simulink model "TBRe19_ECU_SequentialTests"  (R2017b)
settings: Solver=FixedStepDiscrete  StartTime=0.0  StopTime=inf  FixedStep=0.0001  RelTol=1e-3
PostLoadFcn:
  | model_init();
libraries: simulink x28
(part 14 of 22)

== system TBRe19_ECU_SequentialTests/TSSBrake/Comms_And_Data_Acquisition_Layer/MCU_CAN ==
  note: Overall Functionality:
      | Read CAN messages related to motor control unit (MCU)
  Bus Creator1 : BusCreator  Inputs=4
  CanRx1 : S-Function  FunctionName=NsiCan_Rx_J1939_Ext  Parameters=data_can,channel,msg_name,ident,ident_type,dlc,signals,is_trigger,is_SA_Masked,is_TA_Masked,is_physical,is_canfd  SFunctionDeploymentMode=off  EnableBusSupport=off  mask(MUXlink Can Rx){data_can=1;HIGH_SPEED;500Kbps;No;C:\Users\TBRe-admin\Documents\Database\TBRe19_DBC_190617.dbc;0;;;0;HIGH_SPEED;500Kbps;120 Ohm;C:\Users\TBRe-admin\Documents\Database\TBRe19_DBC_190517.dbc;0;;;0;HIGH_SPEED;1000Kbps;120 Ohm;D:\TOOLS\MUXLINK\R2011b\MUXlink\misc\BASE_CAN_MUXLAB4.dbc;0;;;0;HIGH_SPEED;500Kbps;120 Ohm;D:\TOOLS\MUXLINK\R2011b\MUXlink\misc\j1939_adapt.dbc;0;;;0;HIGH_SPEED;1000Kbps;No;D:\TOOLS\MUXLINK\R2011b\MUXlink\misc\BASE_CAN_MUXLAB4.dbc;0;;, channel=1, msg_name=HS3_Temperature_Feedback, ident=0x191AFF71, ident_type=XTD, dlc=8, signals=DC_Link_Voltage;1;32;-16;0.062500;0.000000;V;MotorTemperature;1;16;-16;1.000000;0.000000;C, is_trigger=0, is_physical=0, is_canfd=0, is_SA_Masked=1, is_TA_Masked=0}
      mask prompts: data_can "data can"; msg_name "msg name"; is_SA_Masked "J1939 SA filtering"; is_TA_Masked "J1939 TA filtering"
      mask help: Receive a frame from a CAN channel.
      mask init:
      | NsiCan_Rx_J1939_Ext_InitializationFcn();
      settings: OpenFcn=NsiCan_Rx_J1939_Ext_OpenFcn();
      mask Help:
      | eval('block=get_param(gcb, ''RTWdata'');')
      | web([docroot '\toolbox\MUXlink\html\blocks/' block.MUXlink_BlockType '.html'])
      mask Callback data_can: NsiCan_Rx_J1939_Ext_ApplyFcn(1);
      mask Callback channel: NsiCan_Rx_J1939_Ext_ApplyFcn(2);
      mask Callback msg_name: NsiCan_Rx_J1939_Ext_ApplyFcn(3);
      mask Callback ident: NsiCan_Rx_J1939_Ext_ApplyFcn(4);
      mask Callback ident_type: NsiCan_Rx_J1939_Ext_ApplyFcn(5);
      mask Callback dlc: NsiCan_Rx_J1939_Ext_ApplyFcn(6);
      mask Callback signals: NsiCan_Rx_J1939_Ext_ApplyFcn(7);
      mask Callback is_trigger: NsiCan_Rx_J1939_Ext_ApplyFcn(8);
      mask Callback is_physical: NsiCan_Rx_J1939_Ext_ApplyFcn(9);
      mask Callback is_canfd: NsiCan_Rx_J1939_Ext_ApplyFcn(10);
      mask Callback is_SA_Masked: NsiCan_Rx_J1939_Ext_ApplyFcn(11);
      mask Callback is_TA_Masked: NsiCan_Rx_J1939_Ext_ApplyFcn(12);
      mask Display: image(imread('nsi.bmp'));text(0.5, 0.3, 'J1939_PGN  HS3_Temperature_Feedbackchannel CAN1', 'horizontalAlignment', 'center', 'verticalAlignment', 'base');plot([0.05 0.05 0.05 0.05 0.05 0.05 0.05 0.05 0.05 0.05]); port_label('output',1, 'DC_Link_Voltage'); port_label('output',2, 'MotorTemperature'); port_label('output',3, 'Status');
  CanRx2 : S-Function  FunctionName=NsiCan_Rx_J1939_Ext  Parameters=data_can,channel,msg_name,ident,ident_type,dlc,signals,is_trigger,is_SA_Masked,is_TA_Masked,is_physical,is_canfd  SFunctionDeploymentMode=off  EnableBusSupport=off  mask(MUXlink Can Rx){data_can=1;HIGH_SPEED;500Kbps;No;C:\Users\TBRe-admin\Documents\Database\TBRe19_DBC_190617.dbc;0;;;0;HIGH_SPEED;500Kbps;120 Ohm;C:\Users\TBRe-admin\Documents\Database\TBRe19_DBC_190517.dbc;0;;;0;HIGH_SPEED;1000Kbps;120 Ohm;D:\TOOLS\MUXLINK\R2011b\MUXlink\misc\BASE_CAN_MUXLAB4.dbc;0;;;0;HIGH_SPEED;500Kbps;120 Ohm;D:\TOOLS\MUXLINK\R2011b\MUXlink\misc\j1939_adapt.dbc;0;;;0;HIGH_SPEED;1000Kbps;No;D:\TOOLS\MUXLINK\R2011b\MUXlink\misc\BASE_CAN_MUXLAB4.dbc;0;;, channel=1, msg_name=HD4_Debug_Temperatures_B, ident=0x192BFF71, ident_type=XTD, dlc=8, signals=Debug_Temps_Heatsink;1;24;8;1.000000;0.000000;degC, is_trigger=0, is_physical=0, is_canfd=0, is_SA_Masked=1, is_TA_Masked=0}
      mask prompts: data_can "data can"; msg_name "msg name"; is_SA_Masked "J1939 SA filtering"; is_TA_Masked "J1939 TA filtering"
      mask help: Receive a frame from a CAN channel.
      mask init:
      | NsiCan_Rx_J1939_Ext_InitializationFcn();
      settings: OpenFcn=NsiCan_Rx_J1939_Ext_OpenFcn();
      mask Help:
      | eval('block=get_param(gcb, ''RTWdata'');')
      | web([docroot '\toolbox\MUXlink\html\blocks/' block.MUXlink_BlockType '.html'])
      mask Callback data_can: NsiCan_Rx_J1939_Ext_ApplyFcn(1);
      mask Callback channel: NsiCan_Rx_J1939_Ext_ApplyFcn(2);
      mask Callback msg_name: NsiCan_Rx_J1939_Ext_ApplyFcn(3);
      mask Callback ident: NsiCan_Rx_J1939_Ext_ApplyFcn(4);
      mask Callback ident_type: NsiCan_Rx_J1939_Ext_ApplyFcn(5);
      mask Callback dlc: NsiCan_Rx_J1939_Ext_ApplyFcn(6);
      mask Callback signals: NsiCan_Rx_J1939_Ext_ApplyFcn(7);
      mask Callback is_trigger: NsiCan_Rx_J1939_Ext_ApplyFcn(8);
      mask Callback is_physical: NsiCan_Rx_J1939_Ext_ApplyFcn(9);
      mask Callback is_canfd: NsiCan_Rx_J1939_Ext_ApplyFcn(10);
      mask Callback is_SA_Masked: NsiCan_Rx_J1939_Ext_ApplyFcn(11);
      mask Callback is_TA_Masked: NsiCan_Rx_J1939_Ext_ApplyFcn(12);
      mask Display: image(imread('nsi.bmp'));text(0.5, 0.3, 'J1939_PGN  HD4_Debug_Temperatures_Bchannel CAN1', 'horizontalAlignment', 'center', 'verticalAlignment', 'base');plot([0.05 0.05 0.05 0.05 0.05 0.05 0.05 0.05 0.05 0.05]); port_label('output',1, 'Debug_Temps_Heatsink'); port_label('output',2, 'Status');
  CanRx3 : S-Function  FunctionName=NsiCan_Rx_J1939_Ext  Parameters=data_can,channel,msg_name,ident,ident_type,dlc,signals,is_trigger,is_SA_Masked,is_TA_Masked,is_physical,is_canfd  SFunctionDeploymentMode=off  EnableBusSupport=off  mask(MUXlink Can Rx){data_can=1;HIGH_SPEED;500Kbps;No;C:\Users\TBRe-admin\Documents\Database\TBRe19_DBC_190617.dbc;0;;;0;HIGH_SPEED;500Kbps;120 Ohm;C:\Users\TBRe-admin\Documents\Database\TBRe19_DBC_190517.dbc;0;;;0;HIGH_SPEED;1000Kbps;120 Ohm;D:\TOOLS\MUXLINK\R2011b\MUXlink\misc\BASE_CAN_MUXLAB4.dbc;0;;;0;HIGH_SPEED;500Kbps;120 Ohm;D:\TOOLS\MUXLINK\R2011b\MUXlink\misc\j1939_adapt.dbc;0;;;0;HIGH_SPEED;1000Kbps;No;D:\TOOLS\MUXLINK\R2011b\MUXlink\misc\BASE_CAN_MUXLAB4.dbc;0;;, channel=1, msg_name=HS1_Torque_Feedback, ident=0x1918FF71, ident_type=XTD, dlc=8, signals=Speed_Measured;1;16;-16;1.000000;0.000000;RPM, is_trigger=0, is_physical=0, is_canfd=0, is_SA_Masked=1, is_TA_Masked=0}
      mask prompts: data_can "data can"; msg_name "msg name"; is_SA_Masked "J1939 SA filtering"; is_TA_Masked "J1939 TA filtering"
      mask help: Receive a frame from a CAN channel.
      mask init:
      | NsiCan_Rx_J1939_Ext_InitializationFcn();
      settings: OpenFcn=NsiCan_Rx_J1939_Ext_OpenFcn();
      mask Help:
      | eval('block=get_param(gcb, ''RTWdata'');')
      | web([docroot '\toolbox\MUXlink\html\blocks/' block.MUXlink_BlockType '.html'])
      mask Callback data_can: NsiCan_Rx_J1939_Ext_ApplyFcn(1);
      mask Callback channel: NsiCan_Rx_J1939_Ext_ApplyFcn(2);
      mask Callback msg_name: NsiCan_Rx_J1939_Ext_ApplyFcn(3);
      mask Callback ident: NsiCan_Rx_J1939_Ext_ApplyFcn(4);
      mask Callback ident_type: NsiCan_Rx_J1939_Ext_ApplyFcn(5);
      mask Callback dlc: NsiCan_Rx_J1939_Ext_ApplyFcn(6);
      mask Callback signals: NsiCan_Rx_J1939_Ext_ApplyFcn(7);
      mask Callback is_trigger: NsiCan_Rx_J1939_Ext_ApplyFcn(8);
      mask Callback is_physical: NsiCan_Rx_J1939_Ext_ApplyFcn(9);
      mask Callback is_canfd: NsiCan_Rx_J1939_Ext_ApplyFcn(10);
      mask Callback is_SA_Masked: NsiCan_Rx_J1939_Ext_ApplyFcn(11);
      mask Callback is_TA_Masked: NsiCan_Rx_J1939_Ext_ApplyFcn(12);
      mask Display: image(imread('nsi.bmp'));text(0.5, 0.3, 'J1939_PGN  HS1_Torque_Feedbackchannel CAN1', 'horizontalAlignment', 'center', 'verticalAlignment', 'base');plot([0.05 0.05 0.05 0.05 0.05 0.05 0.05 0.05 0.05 0.05]); port_label('output',1, 'Speed_Measured'); port_label('output',2, 'Status');
  HAL_MCU : Outport
  wires:
  Bus Creator1/1 -> HAL_MCU/1  "HAL_MCU"
  CanRx1/1 -> Bus Creator1/1  "MCU_Voltage"
  CanRx1/2 -> Bus Creator1/2  "Motor_Temp"
  CanRx2/1 -> Bus Creator1/3  "MCU_Temp"
  CanRx3/1 -> Bus Creator1/4  "Motor_Speed"

== system TBRe19_ECU_SequentialTests/TSSBrake/Comms_And_Data_Acquisition_Layer/SENSOR_CAN ==
  note: Overall Functionality:
      | Read CAN messages related to vehicle sensors
  Bus Creator3 : BusCreator  Inputs=9
  CanRx1 : S-Function  FunctionName=NsiCan_Rx_Ext  Parameters=data_can,channel,msg_name,ident,ident_type,dlc,signals,is_trigger,is_physical,is_canfd,is_rxgw  SFunctionDeploymentMode=off  EnableBusSupport=off  mask(MUXlink Can Rx){data_can=1;HIGH_SPEED;500Kbps;No;C:\Users\TBRe-admin\Documents\Database\TBRe19_DBC_190617.dbc;0;;;0;HIGH_SPEED;500Kbps;120 Ohm;C:\Users\TBRe-admin\Documents\Database\TBRe19_DBC_190517.dbc;0;;;0;HIGH_SPEED;1000Kbps;120 Ohm;D:\TOOLS\MUXLINK\R2011b\MUXlink\misc\BASE_CAN_MUXLAB4.dbc;0;;;0;HIGH_SPEED;500Kbps;120 Ohm;D:\TOOLS\MUXLINK\R2011b\MUXlink\misc\j1939_adapt.dbc;0;;;0;HIGH_SPEED;1000Kbps;No;D:\TOOLS\MUXLINK\R2011b\MUXlink\misc\BASE_CAN_MUXLAB4.dbc;0;;, channel=1, msg_name=Front_Wheel_Speeds, ident=0x502, ident_type=STD, dlc=6, signals=Front_Left_Wheel_Speed;1;16;16;0.100000;0.000000;rpm;Front_Right_Wheel_Speed;1;0;16;0.100000;0.000000;rpm;Vehicle_Speed;1;32;16;0.010000;0.000000;_, is_trigger=0, is_physical=0, is_canfd=0, is_rxgw=0}
      mask prompts: data_can "data can"; msg_name "msg name"
      mask help: Receive a frame from a CAN channel.
      mask init:
      | NsiCan_Rx_Ext_InitializationFcn();
      settings: OpenFcn=NsiCan_Rx_Ext_OpenFcn();
      mask Help:
      | eval('block=get_param(gcb, ''RTWdata'');')
      | web([docroot '\toolbox\MUXlink\html\blocks/' block.MUXlink_BlockType '.html'])
      mask Callback data_can: NsiCan_Rx_Ext_ApplyFcn(1);
      mask Callback channel: NsiCan_Rx_Ext_ApplyFcn(2);
      mask Callback msg_name: NsiCan_Rx_Ext_ApplyFcn(3);
      mask Callback ident: NsiCan_Rx_Ext_ApplyFcn(4);
      mask Callback ident_type: NsiCan_Rx_Ext_ApplyFcn(5);
      mask Callback dlc: NsiCan_Rx_Ext_ApplyFcn(6);
      mask Callback signals: NsiCan_Rx_Ext_ApplyFcn(7);
      mask Callback is_trigger: NsiCan_Rx_Ext_ApplyFcn(8);
      mask Callback is_physical: NsiCan_Rx_Ext_ApplyFcn(9);
      mask Callback is_canfd: NsiCan_Rx_Ext_ApplyFcn(10);
      mask Callback is_rxgw: NsiCan_Rx_Ext_ApplyFcn(11);
      mask Display: image(imread('nsi.bmp'));text(0.5, 0.3, 'RX_Front_Wheel_Speeds_CAN1', 'horizontalAlignment', 'center', 'verticalAlignment', 'base');plot([0.05 0.05 0.05 0.05 0.05 0.05 0.05 0.05 0.05 0.05]); port_label('output',1, 'Front_Left_Wheel_Speed'); port_label('output',2, 'Front_Right_Wheel_Speed'); port_label('output',3, 'Vehicle_Speed'); port_label('output',4, 'Status');
  CanRx2 : S-Function  FunctionName=NsiCan_Rx_Ext  Parameters=data_can,channel,msg_name,ident,ident_type,dlc,signals,is_trigger,is_physical,is_canfd,is_rxgw  SFunctionDeploymentMode=off  EnableBusSupport=off  mask(MUXlink Can Rx){data_can=1;HIGH_SPEED;500Kbps;No;C:\Users\TBRe-admin\Documents\Database\TBRe19_DBC_190617.dbc;0;;;0;HIGH_SPEED;500Kbps;120 Ohm;C:\Users\TBRe-admin\Documents\Database\TBRe19_DBC_190517.dbc;0;;;0;HIGH_SPEED;1000Kbps;120 Ohm;D:\TOOLS\MUXLINK\R2011b\MUXlink\misc\BASE_CAN_MUXLAB4.dbc;0;;;0;HIGH_SPEED;500Kbps;120 Ohm;D:\TOOLS\MUXLINK\R2011b\MUXlink\misc\j1939_adapt.dbc;0;;;0;HIGH_SPEED;1000Kbps;No;D:\TOOLS\MUXLINK\R2011b\MUXlink\misc\BASE_CAN_MUXLAB4.dbc;0;;, channel=1, msg_name=Rear_Wheel_Speed, ident=0x501, ident_type=STD, dlc=6, signals=Rear_Left_Wheel_Speed;1;16;16;0.100000;0.000000;rpm;Rear_Right_Wheel_Speed;1;0;16;0.100000;0.000000;rpm;Rear_Wheel_Speed;1;32;16;0.010000;0.000000;km/h, is_trigger=0, is_physical=0, is_canfd=0, is_rxgw=0}
      mask prompts: data_can "data can"; msg_name "msg name"
      mask help: Receive a frame from a CAN channel.
      mask init:
      | NsiCan_Rx_Ext_InitializationFcn();
      settings: OpenFcn=NsiCan_Rx_Ext_OpenFcn();
      mask Help:
      | eval('block=get_param(gcb, ''RTWdata'');')
      | web([docroot '\toolbox\MUXlink\html\blocks/' block.MUXlink_BlockType '.html'])
      mask Callback data_can: NsiCan_Rx_Ext_ApplyFcn(1);
      mask Callback channel: NsiCan_Rx_Ext_ApplyFcn(2);
      mask Callback msg_name: NsiCan_Rx_Ext_ApplyFcn(3);
      mask Callback ident: NsiCan_Rx_Ext_ApplyFcn(4);
      mask Callback ident_type: NsiCan_Rx_Ext_ApplyFcn(5);
      mask Callback dlc: NsiCan_Rx_Ext_ApplyFcn(6);
      mask Callback signals: NsiCan_Rx_Ext_ApplyFcn(7);
      mask Callback is_trigger: NsiCan_Rx_Ext_ApplyFcn(8);
      mask Callback is_physical: NsiCan_Rx_Ext_ApplyFcn(9);
      mask Callback is_canfd: NsiCan_Rx_Ext_ApplyFcn(10);
      mask Callback is_rxgw: NsiCan_Rx_Ext_ApplyFcn(11);
      mask Display: image(imread('nsi.bmp'));text(0.5, 0.3, 'RX_Rear_Wheel_Speed_CAN1', 'horizontalAlignment', 'center', 'verticalAlignment', 'base');plot([0.05 0.05 0.05 0.05 0.05 0.05 0.05 0.05 0.05 0.05]); port_label('output',1, 'Rear_Left_Wheel_Speed'); port_label('output',2, 'Rear_Right_Wheel_Speed'); port_label('output',3, 'Rear_Wheel_Speed'); port_label('output',4, 'Status');
  CanRx5 : S-Function  FunctionName=NsiCan_Rx_Ext  Parameters=data_can,channel,msg_name,ident,ident_type,dlc,signals,is_trigger,is_physical,is_canfd,is_rxgw  SFunctionDeploymentMode=off  EnableBusSupport=off  mask(MUXlink Can Rx){data_can=1;HIGH_SPEED;500Kbps;No;C:\Users\TBRe-admin\Documents\Database\TBRe19_DBC_190617.dbc;0;;;0;HIGH_SPEED;500Kbps;120 Ohm;C:\Users\TBRe-admin\Documents\Database\TBRe19_DBC_190517.dbc;0;;;0;HIGH_SPEED;1000Kbps;120 Ohm;D:\TOOLS\MUXLINK\R2011b\MUXlink\misc\BASE_CAN_MUXLAB4.dbc;0;;;0;HIGH_SPEED;500Kbps;120 Ohm;D:\TOOLS\MUXLINK\R2011b\MUXlink\misc\j1939_adapt.dbc;0;;;0;HIGH_SPEED;1000Kbps;No;D:\TOOLS\MUXLINK\R2011b\MUXlink\misc\BASE_CAN_MUXLAB4.dbc;0;;, channel=1, msg_name=SteeringWheelSensor, ident=0x234, ident_type=STD, dlc=5, signals=Acc_Angle;1;0;-16;0.100000;0.000000;Degrees, is_trigger=0, is_physical=0, is_canfd=0, is_rxgw=0}
      mask prompts: data_can "data can"; msg_name "msg name"
      mask help: Receive a frame from a CAN channel.
      mask init:
      | NsiCan_Rx_Ext_InitializationFcn();
      settings: OpenFcn=NsiCan_Rx_Ext_OpenFcn();
      mask Help:
      | eval('block=get_param(gcb, ''RTWdata'');')
      | web([docroot '\toolbox\MUXlink\html\blocks/' block.MUXlink_BlockType '.html'])
      mask Callback data_can: NsiCan_Rx_Ext_ApplyFcn(1);
      mask Callback channel: NsiCan_Rx_Ext_ApplyFcn(2);
      mask Callback msg_name: NsiCan_Rx_Ext_ApplyFcn(3);
      mask Callback ident: NsiCan_Rx_Ext_ApplyFcn(4);
      mask Callback ident_type: NsiCan_Rx_Ext_ApplyFcn(5);
      mask Callback dlc: NsiCan_Rx_Ext_ApplyFcn(6);
      mask Callback signals: NsiCan_Rx_Ext_ApplyFcn(7);
      mask Callback is_trigger: NsiCan_Rx_Ext_ApplyFcn(8);
      mask Callback is_physical: NsiCan_Rx_Ext_ApplyFcn(9);
      mask Callback is_canfd: NsiCan_Rx_Ext_ApplyFcn(10);
      mask Callback is_rxgw: NsiCan_Rx_Ext_ApplyFcn(11);
      mask Display: image(imread('nsi.bmp'));text(0.5, 0.3, 'RX_SteeringWheelSensor_CAN1', 'horizontalAlignment', 'center', 'verticalAlignment', 'base');plot([0.05 0.05 0.05 0.05 0.05 0.05 0.05 0.05 0.05 0.05]); port_label('output',1, 'Acc_Angle'); port_label('output',2, 'Status');
  CanRx8 : S-Function  FunctionName=NsiCan_Rx_Ext  Parameters=data_can,channel,msg_name,ident,ident_type,dlc,signals,is_trigger,is_physical,is_canfd,is_rxgw  SFunctionDeploymentMode=off  EnableBusSupport=off  mask(MUXlink Can Rx){data_can=1;HIGH_SPEED;500Kbps;No;C:\Users\TBRe-admin\Documents\Database\TBRe19_DBC_190617.dbc;0;;;0;HIGH_SPEED;500Kbps;120 Ohm;C:\Users\TBRe-admin\Documents\Database\TBRe19_DBC_190517.dbc;0;;;0;HIGH_SPEED;1000Kbps;120 Ohm;D:\TOOLS\MUXLINK\R2011b\MUXlink\misc\BASE_CAN_MUXLAB4.dbc;0;;;0;HIGH_SPEED;500Kbps;120 Ohm;D:\TOOLS\MUXLINK\R2011b\MUXlink\misc\j1939_adapt.dbc;0;;;0;HIGH_SPEED;1000Kbps;No;D:\TOOLS\MUXLINK\R2011b\MUXlink\misc\BASE_CAN_MUXLAB4.dbc;0;;, channel=1, msg_name=AccelerometerY, ident=0x174, ident_type=STD, dlc=8, signals=Acc_Yaw;1;0;16;0.005000;0.000000;_, is_trigger=0, is_physical=0, is_canfd=0, is_rxgw=0}
      mask prompts: data_can "data can"; msg_name "msg name"
      mask help: Receive a frame from a CAN channel.
      mask init:
      | NsiCan_Rx_Ext_InitializationFcn();
      settings: OpenFcn=NsiCan_Rx_Ext_OpenFcn();
      mask Help:
      | eval('block=get_param(gcb, ''RTWdata'');')
      | web([docroot '\toolbox\MUXlink\html\blocks/' block.MUXlink_BlockType '.html'])
      mask Callback data_can: NsiCan_Rx_Ext_ApplyFcn(1);
      mask Callback channel: NsiCan_Rx_Ext_ApplyFcn(2);
      mask Callback msg_name: NsiCan_Rx_Ext_ApplyFcn(3);
      mask Callback ident: NsiCan_Rx_Ext_ApplyFcn(4);
      mask Callback ident_type: NsiCan_Rx_Ext_ApplyFcn(5);
      mask Callback dlc: NsiCan_Rx_Ext_ApplyFcn(6);
      mask Callback signals: NsiCan_Rx_Ext_ApplyFcn(7);
      mask Callback is_trigger: NsiCan_Rx_Ext_ApplyFcn(8);
      mask Callback is_physical: NsiCan_Rx_Ext_ApplyFcn(9);
      mask Callback is_canfd: NsiCan_Rx_Ext_ApplyFcn(10);
      mask Callback is_rxgw: NsiCan_Rx_Ext_ApplyFcn(11);
      mask Display: image(imread('nsi.bmp'));text(0.5, 0.3, 'RX_AccelerometerY_CAN1', 'horizontalAlignment', 'center', 'verticalAlignment', 'base');plot([0.05 0.05 0.05 0.05 0.05 0.05 0.05 0.05 0.05 0.05]); port_label('output',1, 'Acc_Yaw'); port_label('output',2, 'Status');
  CanRx9 : S-Function  FunctionName=NsiCan_Rx_Ext  Parameters=data_can,channel,msg_name,ident,ident_type,dlc,signals,is_trigger,is_physical,is_canfd,is_rxgw  SFunctionDeploymentMode=off  EnableBusSupport=off  mask(MUXlink Can Rx){data_can=1;HIGH_SPEED;500Kbps;No;C:\Users\TBRe-admin\Documents\Database\TBRe19_DBC_190620.dbc;0;;;0;HIGH_SPEED;500Kbps;120 Ohm;C:\Users\TBRe-admin\Documents\Database\TBRe19_DBC_190517.dbc;0;;;0;HIGH_SPEED;1000Kbps;120 Ohm;D:\TOOLS\MUXLINK\R2011b\MUXlink\misc\BASE_CAN_MUXLAB4.dbc;0;;;0;HIGH_SPEED;500Kbps;120 Ohm;D:\TOOLS\MUXLINK\R2011b\MUXlink\misc\j1939_adapt.dbc;0;;;0;HIGH_SPEED;1000Kbps;No;D:\TOOLS\MUXLINK\R2011b\MUXlink\misc\BASE_CAN_MUXLAB4.dbc;0;;, channel=1, msg_name=Shutdown_Data, ident=0x705, ident_type=STD, dlc=3, signals=Fault_CarShutdown;1;0;1;1.000000;0.000000;_, is_trigger=0, is_physical=0, is_canfd=0, is_rxgw=0}
      mask prompts: data_can "data can"; msg_name "msg name"
      mask help: Receive a frame from a CAN channel.
      mask init:
      | NsiCan_Rx_Ext_InitializationFcn();
      settings: OpenFcn=NsiCan_Rx_Ext_OpenFcn();
      mask Help:
      | eval('block=get_param(gcb, ''RTWdata'');')
      | web([docroot '\toolbox\MUXlink\html\blocks/' block.MUXlink_BlockType '.html'])
      mask Callback data_can: NsiCan_Rx_Ext_ApplyFcn(1);
      mask Callback channel: NsiCan_Rx_Ext_ApplyFcn(2);
      mask Callback msg_name: NsiCan_Rx_Ext_ApplyFcn(3);
      mask Callback ident: NsiCan_Rx_Ext_ApplyFcn(4);
      mask Callback ident_type: NsiCan_Rx_Ext_ApplyFcn(5);
      mask Callback dlc: NsiCan_Rx_Ext_ApplyFcn(6);
      mask Callback signals: NsiCan_Rx_Ext_ApplyFcn(7);
      mask Callback is_trigger: NsiCan_Rx_Ext_ApplyFcn(8);
      mask Callback is_physical: NsiCan_Rx_Ext_ApplyFcn(9);
      mask Callback is_canfd: NsiCan_Rx_Ext_ApplyFcn(10);
      mask Callback is_rxgw: NsiCan_Rx_Ext_ApplyFcn(11);
      mask Display: image(imread('nsi.bmp'));text(0.5, 0.3, 'RX_Shutdown_Data_CAN1', 'horizontalAlignment', 'center', 'verticalAlignment', 'base');plot([0.05 0.05 0.05 0.05 0.05 0.05 0.05 0.05 0.05 0.05]); port_label('output',1, 'Fault_CarShutdown'); port_label('output',2, 'Status');
  Sensor_Data : Outport
  wires:
  CanRx5/2 -> ?
  CanRx1/4 -> ?
  CanRx2/4 -> ?
  CanRx8/2 -> ?
  CanRx9/2 -> ?
  CanRx9/1 -> Bus Creator3/9  "Shutdown_Error"
  CanRx2/2 -> Bus Creator3/5  "Rear_Right_Wheel_Speed"
  CanRx2/3 -> Bus Creator3/6  "Rear_Wheel_Speed"
  CanRx5/1 -> Bus Creator3/7  "Steering_Angle"
  CanRx8/1 -> Bus Creator3/8  "Yaw"
  CanRx1/1 -> Bus Creator3/1  "Front_Left_Wheel_Speed"
  CanRx1/2 -> Bus Creator3/2  "Front_Right_Wheel_Speed"
  CanRx2/1 -> Bus Creator3/4  "Rear_Left_Wheel_Speed"
  Bus Creator3/1 -> Sensor_Data/1  "Sensor_Data"
  CanRx1/3 -> Bus Creator3/3  "Vehicle_Speed"

== system TBRe19_ECU_SequentialTests/TSSBrake/Comms_And_Data_Output_Layer/Hardwired_Ouputs ==
  note: Turns the MCU on
  PostPL_Data : Inport
  Bus Selector : BusSelector  OutputSignals=Hardwired_Peripherals.TSS
  DigitalOutput2 : S-Function  FunctionName=NsiIo_DigitalOutput  Parameters=channel,side,feedback  SFunctionDeploymentMode=off  EnableBusSupport=off  mask(MUXlink I/O Digital Output){channel=1, side=High, feedback=off}
      mask prompts: channel "Channel ?"; side "Side ?"; feedback "With feedback ?"
      mask help: Write Digital Output onto I/O channel.
      mask init:
      | NsiIo_DigitalOutput_InitializationFcn();
      settings: OpenFcn=NsiIo_DigitalOutput_OpenFcn();
      mask Help:
      | eval('block=get_param(gcb, ''RTWdata'');')
      | web([docroot '\toolbox\MUXlink\html\blocks/' block.MUXlink_BlockType '.html'])
      mask Callback channel: NsiIo_DigitalOutput_ApplyFcn(1);
      mask TypeOptions side: High | Low
      mask Callback side: NsiIo_DigitalOutput_ApplyFcn(2);
      mask Callback feedback: NsiIo_DigitalOutput_ApplyFcn(3);
      mask Display: image(imread('nsi.bmp'));text(0.5, 0.2, 'DigitalOutput_1', 'horizontalAlignment', 'center', 'verticalAlignment', 'base');plot([0.05 0.05 0.05 0.05 0.05 0.05 0.05 0.05 0.05 0.05]);port_label('input', 1, 'G2 : High Side');
  wires:
  PostPL_Data/1 -> Bus Selector/1
  Bus Selector/1 -> DigitalOutput2/1  "<TSS>"

== system TBRe19_ECU_SequentialTests/TSSBrake/Post_Processing_Layer/Hardwired_Peripherals ==
  note: Talk to Wilkins about when you want pump and fans
      | power switching between Vicor and LV to occur
  VFL_Data : Inport
  Bus Creator : BusCreator  Inputs=7
  Bus Selector3 : BusSelector  OutputSignals=VOM_Data.TSS
  Hardwired_Peripherals : Outport
  wires:
  VFL_Data/1 -> Bus Selector3/1
  Bus Selector3/1 -> Bus Creator/3  "<TSS>"
  Bus Creator/1 -> Hardwired_Peripherals/1  "Hardwired_Peripherals"

== system TBRe19_ECU_SequentialTests/TSSBrake/Vehicle_Functionality_Layer/Vehicle_Operation_Mode ==
  PrePL_Data : Inport
  Bus Creator : BusCreator  Inputs=5
  TSS : Subsystem
  VOM_Data : Outport
  wires:
  Bus Creator/1 -> VOM_Data/1  "Vehicle_Operation_Data"
  PrePL_Data/1 -> TSS/1(PrePL_Data)
  TSS/1(TS_StartUp) -> Bus Creator/5  "TSS"

== system TBRe19_ECU_SequentialTests/DriveFunction/Comms_And_Data_Acquisition_Layer/Hardwired_Inputs_2019/AIRs ==
  DigitalInput : S-Function  FunctionName=NsiIo_DigitalInput  Parameters=channel,is_trigger,typeof_trigger,is_wakeup,wakeup_level  SFunctionDeploymentMode=off  EnableBusSupport=off  mask(MUXlink I/O Digital Input){channel=1, is_trigger=off, typeof_trigger=Either, is_wakeup=off, wakeup_level=Low level}
      mask prompts: channel "Channel ?"; is_trigger "Trigger ?"; typeof_trigger "Type of Trigger ?"; is_wakeup "Wake-up ?"; wakeup_level "Wake-up level ?"
      mask help: Read digital input from I/O channel.
      mask init:
      | NsiIo_DigitalInput_InitializationFcn();
      settings: OpenFcn=NsiIo_DigitalInput_OpenFcn();
      mask Help:
      | eval('block=get_param(gcb, ''RTWdata'');')
      | web([docroot '\toolbox\MUXlink\html\blocks/' block.MUXlink_BlockType '.html'])
      mask Callback channel: NsiIo_DigitalInput_ApplyFcn(1);
      mask Callback is_trigger: NsiIo_DigitalInput_ApplyFcn(2);
      mask TypeOptions typeof_trigger: Rising | Falling | Either
      mask Callback typeof_trigger: NsiIo_DigitalInput_ApplyFcn(3);
      mask Callback is_wakeup: NsiIo_DigitalInput_ApplyFcn(4);
      mask TypeOptions wakeup_level: Low level | High level
      mask Callback wakeup_level: NsiIo_DigitalInput_ApplyFcn(5);
      mask Display: image(imread('nsi.bmp'));text(0.5, 0.2, 'DigitalInput_1', 'horizontalAlignment', 'center', 'verticalAlignment', 'base');plot([0.05 0.05 0.05 0.05 0.05 0.05 0.05 0.05 0.05 0.05]);port_label('output', 1, 'Ground : A1');
  DigitalInput5 : S-Function  FunctionName=NsiIo_DigitalInput  Parameters=channel,is_trigger,typeof_trigger,is_wakeup,wakeup_level  SFunctionDeploymentMode=off  EnableBusSupport=off  mask(MUXlink I/O Digital Input){channel=2, is_trigger=off, typeof_trigger=Either, is_wakeup=off, wakeup_level=Low level}
      mask prompts: channel "Channel ?"; is_trigger "Trigger ?"; typeof_trigger "Type of Trigger ?"; is_wakeup "Wake-up ?"; wakeup_level "Wake-up level ?"
      mask help: Read digital input from I/O channel.
      mask init:
      | NsiIo_DigitalInput_InitializationFcn();
      settings: OpenFcn=NsiIo_DigitalInput_OpenFcn();
      mask Help:
      | eval('block=get_param(gcb, ''RTWdata'');')
      | web([docroot '\toolbox\MUXlink\html\blocks/' block.MUXlink_BlockType '.html'])
      mask Callback channel: NsiIo_DigitalInput_ApplyFcn(1);
      mask Callback is_trigger: NsiIo_DigitalInput_ApplyFcn(2);
      mask TypeOptions typeof_trigger: Rising | Falling | Either
      mask Callback typeof_trigger: NsiIo_DigitalInput_ApplyFcn(3);
      mask Callback is_wakeup: NsiIo_DigitalInput_ApplyFcn(4);
      mask TypeOptions wakeup_level: Low level | High level
      mask Callback wakeup_level: NsiIo_DigitalInput_ApplyFcn(5);
      mask Display: image(imread('nsi.bmp'));text(0.5, 0.2, 'DigitalInput_2', 'horizontalAlignment', 'center', 'verticalAlignment', 'base');plot([0.05 0.05 0.05 0.05 0.05 0.05 0.05 0.05 0.05 0.05]);port_label('output', 1, 'Ground : A2');
  UsbTx1 : S-Function  FunctionName=NsiUsb_Tx  Parameters=signame,resolution,offset,unite  SFunctionDeploymentMode=off  EnableBusSupport=off  mask(MUXlink Usb Tx){signame=AIRLow, resolution=1, offset=0, unite=Bool}
      mask prompts: signame "Signal name ?"; resolution "Resolution ?"; offset "Offset ?"; unite "Unit ?"
      mask help: Transmit a frame on the USB Channel.
      mask init:
      | NsiUsb_Tx_InitializationFcn();
      settings: OpenFcn=NsiUsb_Tx_OpenFcn();
      mask Help:
      | eval('block=get_param(gcb, ''RTWdata'');')
      | web([docroot '\toolbox\MUXlink\html\blocks/' block.MUXlink_BlockType '.html'])
      mask Callback signame: NsiUsb_Tx_ApplyFcn(1);
      mask Callback resolution: NsiUsb_Tx_ApplyFcn(2);
      mask Callback offset: NsiUsb_Tx_ApplyFcn(3);
      mask Callback unite: NsiUsb_Tx_ApplyFcn(4);
      mask Display: image(imread('nsi.bmp'));text(0.5, 0.2, 'USB Tx', 'horizontalAlignment', 'center', 'verticalAlignment', 'base');plot([0.05 0.05 0.05 0.05 0.05 0.05 0.05 0.05 0.05 0.05]);port_label('input',1, 'AIRLow');
  UsbTx2 : S-Function  FunctionName=NsiUsb_Tx  Parameters=signame,resolution,offset,unite  SFunctionDeploymentMode=off  EnableBusSupport=off  mask(MUXlink Usb Tx){signame=AIRHigh, resolution=1, offset=0, unite=Bool}
      mask prompts: signame "Signal name ?"; resolution "Resolution ?"; offset "Offset ?"; unite "Unit ?"
      mask help: Transmit a frame on the USB Channel.
      mask init:
      | NsiUsb_Tx_InitializationFcn();
      settings: OpenFcn=NsiUsb_Tx_OpenFcn();
      mask Help:
      | eval('block=get_param(gcb, ''RTWdata'');')
      | web([docroot '\toolbox\MUXlink\html\blocks/' block.MUXlink_BlockType '.html'])
      mask Callback signame: NsiUsb_Tx_ApplyFcn(1);
      mask Callback resolution: NsiUsb_Tx_ApplyFcn(2);
      mask Callback offset: NsiUsb_Tx_ApplyFcn(3);
      mask Callback unite: NsiUsb_Tx_ApplyFcn(4);
      mask Display: image(imread('nsi.bmp'));text(0.5, 0.2, 'USB Tx', 'horizontalAlignment', 'center', 'verticalAlignment', 'base');plot([0.05 0.05 0.05 0.05 0.05 0.05 0.05 0.05 0.05 0.05]);port_label('input',1, 'AIRHigh');
  AIRLow : Outport
  AIRHigh : Outport  Port=2
  wires:
  DigitalInput/1 -> UsbTx1/1, AIRLow/1  "AIRLow"
  DigitalInput5/1 -> UsbTx2/1, AIRHigh/1  "AIRHigh"

== system TBRe19_ECU_SequentialTests/DriveFunction/Comms_And_Data_Acquisition_Layer/Hardwired_Inputs_2019/BMS ==
  DigitalInput1 : S-Function  FunctionName=NsiIo_DigitalInput  Parameters=channel,is_trigger,typeof_trigger,is_wakeup,wakeup_level  SFunctionDeploymentMode=off  EnableBusSupport=off  mask(MUXlink I/O Digital Input){channel=16, is_trigger=off, typeof_trigger=Either, is_wakeup=off, wakeup_level=Low level}
      mask prompts: channel "Channel ?"; is_trigger "Trigger ?"; typeof_trigger "Type of Trigger ?"; is_wakeup "Wake-up ?"; wakeup_level "Wake-up level ?"
      mask help: Read digital input from I/O channel.
      mask init:
      | NsiIo_DigitalInput_InitializationFcn();
      settings: OpenFcn=NsiIo_DigitalInput_OpenFcn();
      mask Help:
      | eval('block=get_param(gcb, ''RTWdata'');')
      | web([docroot '\toolbox\MUXlink\html\blocks/' block.MUXlink_BlockType '.html'])
      mask Callback channel: NsiIo_DigitalInput_ApplyFcn(1);
      mask Callback is_trigger: NsiIo_DigitalInput_ApplyFcn(2);
      mask TypeOptions typeof_trigger: Rising | Falling | Either
      mask Callback typeof_trigger: NsiIo_DigitalInput_ApplyFcn(3);
      mask Callback is_wakeup: NsiIo_DigitalInput_ApplyFcn(4);
      mask TypeOptions wakeup_level: Low level | High level
      mask Callback wakeup_level: NsiIo_DigitalInput_ApplyFcn(5);
      mask Display: image(imread('nsi.bmp'));text(0.5, 0.2, 'DigitalInput_16', 'horizontalAlignment', 'center', 'verticalAlignment', 'base');plot([0.05 0.05 0.05 0.05 0.05 0.05 0.05 0.05 0.05 0.05]);port_label('output', 1, 'Battery : H2');
  DigitalInput2 : S-Function  FunctionName=NsiIo_DigitalInput  Parameters=channel,is_trigger,typeof_trigger,is_wakeup,wakeup_level  SFunctionDeploymentMode=off  EnableBusSupport=off  mask(MUXlink I/O Digital Input){channel=17, is_trigger=off, typeof_trigger=Either, is_wakeup=off, wakeup_level=Low level}
      mask prompts: channel "Channel ?"; is_trigger "Trigger ?"; typeof_trigger "Type of Trigger ?"; is_wakeup "Wake-up ?"; wakeup_level "Wake-up level ?"
      mask help: Read digital input from I/O channel.
      mask init:
      | NsiIo_DigitalInput_InitializationFcn();
      settings: OpenFcn=NsiIo_DigitalInput_OpenFcn();
      mask Help:
      | eval('block=get_param(gcb, ''RTWdata'');')
      | web([docroot '\toolbox\MUXlink\html\blocks/' block.MUXlink_BlockType '.html'])
      mask Callback channel: NsiIo_DigitalInput_ApplyFcn(1);
      mask Callback is_trigger: NsiIo_DigitalInput_ApplyFcn(2);
      mask TypeOptions typeof_trigger: Rising | Falling | Either
      mask Callback typeof_trigger: NsiIo_DigitalInput_ApplyFcn(3);
      mask Callback is_wakeup: NsiIo_DigitalInput_ApplyFcn(4);
      mask TypeOptions wakeup_level: Low level | High level
      mask Callback wakeup_level: NsiIo_DigitalInput_ApplyFcn(5);
      mask Display: image(imread('nsi.bmp'));text(0.5, 0.2, 'DigitalInput_17', 'horizontalAlignment', 'center', 'verticalAlignment', 'base');plot([0.05 0.05 0.05 0.05 0.05 0.05 0.05 0.05 0.05 0.05]);port_label('output', 1, 'Battery : H3');
  DigitalInput6 : S-Function  FunctionName=NsiIo_DigitalInput  Parameters=channel,is_trigger,typeof_trigger,is_wakeup,wakeup_level  SFunctionDeploymentMode=off  EnableBusSupport=off  mask(MUXlink I/O Digital Input){channel=18, is_trigger=off, typeof_trigger=Either, is_wakeup=off, wakeup_level=Low level}
      mask prompts: channel "Channel ?"; is_trigger "Trigger ?"; typeof_trigger "Type of Trigger ?"; is_wakeup "Wake-up ?"; wakeup_level "Wake-up level ?"
      mask help: Read digital input from I/O channel.
      mask init:
      | NsiIo_DigitalInput_InitializationFcn();
      settings: OpenFcn=NsiIo_DigitalInput_OpenFcn();
      mask Help:
      | eval('block=get_param(gcb, ''RTWdata'');')
      | web([docroot '\toolbox\MUXlink\html\blocks/' block.MUXlink_BlockType '.html'])
      mask Callback channel: NsiIo_DigitalInput_ApplyFcn(1);
      mask Callback is_trigger: NsiIo_DigitalInput_ApplyFcn(2);
      mask TypeOptions typeof_trigger: Rising | Falling | Either
      mask Callback typeof_trigger: NsiIo_DigitalInput_ApplyFcn(3);
      mask Callback is_wakeup: NsiIo_DigitalInput_ApplyFcn(4);
      mask TypeOptions wakeup_level: Low level | High level
      mask Callback wakeup_level: NsiIo_DigitalInput_ApplyFcn(5);
      mask Display: image(imread('nsi.bmp'));text(0.5, 0.2, 'DigitalInput_18', 'horizontalAlignment', 'center', 'verticalAlignment', 'base');plot([0.05 0.05 0.05 0.05 0.05 0.05 0.05 0.05 0.05 0.05]);port_label('output', 1, 'Battery : H4');
  BMS_Multi1 : Outport
  BMS_Multi2 : Outport  Port=2
  BMS_ChargeEnable : Outport  Port=3
  wires:
  DigitalInput6/1 -> BMS_Multi1/1  "BMS_Multi1"
  DigitalInput2/1 -> BMS_ChargeEnable/1  "BMS_ChargeEnable"
  DigitalInput1/1 -> BMS_Multi2/1  "BMS_Multi2"

== system TBRe19_ECU_SequentialTests/DriveFunction/Comms_And_Data_Acquisition_Layer/Hardwired_Inputs_2019/Buttons ==
  DigitalInput1 : S-Function  FunctionName=NsiIo_DigitalInput  Parameters=channel,is_trigger,typeof_trigger,is_wakeup,wakeup_level  SFunctionDeploymentMode=off  EnableBusSupport=off  mask(MUXlink I/O Digital Input){channel=5, is_trigger=off, typeof_trigger=Either, is_wakeup=off, wakeup_level=Low level}
      mask prompts: channel "Channel ?"; is_trigger "Trigger ?"; typeof_trigger "Type of Trigger ?"; is_wakeup "Wake-up ?"; wakeup_level "Wake-up level ?"
      mask help: Read digital input from I/O channel.
      mask init:
      | NsiIo_DigitalInput_InitializationFcn();
      settings: OpenFcn=NsiIo_DigitalInput_OpenFcn();
      mask Help:
      | eval('block=get_param(gcb, ''RTWdata'');')
      | web([docroot '\toolbox\MUXlink\html\blocks/' block.MUXlink_BlockType '.html'])
      mask Callback channel: NsiIo_DigitalInput_ApplyFcn(1);
      mask Callback is_trigger: NsiIo_DigitalInput_ApplyFcn(2);
      mask TypeOptions typeof_trigger: Rising | Falling | Either
      mask Callback typeof_trigger: NsiIo_DigitalInput_ApplyFcn(3);
      mask Callback is_wakeup: NsiIo_DigitalInput_ApplyFcn(4);
      mask TypeOptions wakeup_level: Low level | High level
      mask Callback wakeup_level: NsiIo_DigitalInput_ApplyFcn(5);
      mask Display: image(imread('nsi.bmp'));text(0.5, 0.2, 'DigitalInput_5', 'horizontalAlignment', 'center', 'verticalAlignment', 'base');plot([0.05 0.05 0.05 0.05 0.05 0.05 0.05 0.05 0.05 0.05]);port_label('output', 1, 'Ground : B1');
  DigitalInput2 : S-Function  FunctionName=NsiIo_DigitalInput  Parameters=channel,is_trigger,typeof_trigger,is_wakeup,wakeup_level  SFunctionDeploymentMode=off  EnableBusSupport=off  mask(MUXlink I/O Digital Input){channel=8, is_trigger=off, typeof_trigger=Either, is_wakeup=off, wakeup_level=Low level}
      mask prompts: channel "Channel ?"; is_trigger "Trigger ?"; typeof_trigger "Type of Trigger ?"; is_wakeup "Wake-up ?"; wakeup_level "Wake-up level ?"
      mask help: Read digital input from I/O channel.
      mask init:
      | NsiIo_DigitalInput_InitializationFcn();
      settings: OpenFcn=NsiIo_DigitalInput_OpenFcn();
      mask Help:
      | eval('block=get_param(gcb, ''RTWdata'');')
      | web([docroot '\toolbox\MUXlink\html\blocks/' block.MUXlink_BlockType '.html'])
      mask Callback channel: NsiIo_DigitalInput_ApplyFcn(1);
      mask Callback is_trigger: NsiIo_DigitalInput_ApplyFcn(2);
      mask TypeOptions typeof_trigger: Rising | Falling | Either
      mask Callback typeof_trigger: NsiIo_DigitalInput_ApplyFcn(3);
      mask Callback is_wakeup: NsiIo_DigitalInput_ApplyFcn(4);
      mask TypeOptions wakeup_level: Low level | High level
      mask Callback wakeup_level: NsiIo_DigitalInput_ApplyFcn(5);
      mask Display: image(imread('nsi.bmp'));text(0.5, 0.2, 'DigitalInput_8', 'horizontalAlignment', 'center', 'verticalAlignment', 'base');plot([0.05 0.05 0.05 0.05 0.05 0.05 0.05 0.05 0.05 0.05]);port_label('output', 1, 'Ground : B4');
  DigitalInput3 : S-Function  FunctionName=NsiIo_DigitalInput  Parameters=channel,is_trigger,typeof_trigger,is_wakeup,wakeup_level  SFunctionDeploymentMode=off  EnableBusSupport=off  mask(MUXlink I/O Digital Input){channel=6, is_trigger=off, typeof_trigger=Either, is_wakeup=off, wakeup_level=Low level}
      mask prompts: channel "Channel ?"; is_trigger "Trigger ?"; typeof_trigger "Type of Trigger ?"; is_wakeup "Wake-up ?"; wakeup_level "Wake-up level ?"
      mask help: Read digital input from I/O channel.
      mask init:
      | NsiIo_DigitalInput_InitializationFcn();
      settings: OpenFcn=NsiIo_DigitalInput_OpenFcn();
      mask Help:
      | eval('block=get_param(gcb, ''RTWdata'');')
      | web([docroot '\toolbox\MUXlink\html\blocks/' block.MUXlink_BlockType '.html'])
      mask Callback channel: NsiIo_DigitalInput_ApplyFcn(1);
      mask Callback is_trigger: NsiIo_DigitalInput_ApplyFcn(2);
      mask TypeOptions typeof_trigger: Rising | Falling | Either
      mask Callback typeof_trigger: NsiIo_DigitalInput_ApplyFcn(3);
      mask Callback is_wakeup: NsiIo_DigitalInput_ApplyFcn(4);
      mask TypeOptions wakeup_level: Low level | High level
      mask Callback wakeup_level: NsiIo_DigitalInput_ApplyFcn(5);
      mask Display: image(imread('nsi.bmp'));text(0.5, 0.2, 'DigitalInput_6', 'horizontalAlignment', 'center', 'verticalAlignment', 'base');plot([0.05 0.05 0.05 0.05 0.05 0.05 0.05 0.05 0.05 0.05]);port_label('output', 1, 'Ground : B2');
  DigitalInput4 : S-Function  FunctionName=NsiIo_DigitalInput  Parameters=channel,is_trigger,typeof_trigger,is_wakeup,wakeup_level  SFunctionDeploymentMode=off  EnableBusSupport=off  mask(MUXlink I/O Digital Input){channel=7, is_trigger=off, typeof_trigger=Either, is_wakeup=off, wakeup_level=Low level}
      mask prompts: channel "Channel ?"; is_trigger "Trigger ?"; typeof_trigger "Type of Trigger ?"; is_wakeup "Wake-up ?"; wakeup_level "Wake-up level ?"
      mask help: Read digital input from I/O channel.
      mask init:
      | NsiIo_DigitalInput_InitializationFcn();
      settings: OpenFcn=NsiIo_DigitalInput_OpenFcn();
      mask Help:
      | eval('block=get_param(gcb, ''RTWdata'');')
      | web([docroot '\toolbox\MUXlink\html\blocks/' block.MUXlink_BlockType '.html'])
      mask Callback channel: NsiIo_DigitalInput_ApplyFcn(1);
      mask Callback is_trigger: NsiIo_DigitalInput_ApplyFcn(2);
      mask TypeOptions typeof_trigger: Rising | Falling | Either
      mask Callback typeof_trigger: NsiIo_DigitalInput_ApplyFcn(3);
      mask Callback is_wakeup: NsiIo_DigitalInput_ApplyFcn(4);
      mask TypeOptions wakeup_level: Low level | High level
      mask Callback wakeup_level: NsiIo_DigitalInput_ApplyFcn(5);
      mask Display: image(imread('nsi.bmp'));text(0.5, 0.2, 'DigitalInput_7', 'horizontalAlignment', 'center', 'verticalAlignment', 'base');plot([0.05 0.05 0.05 0.05 0.05 0.05 0.05 0.05 0.05 0.05]);port_label('output', 1, 'Ground : B3');
  DigitalInput5 : S-Function  FunctionName=NsiIo_DigitalInput  Parameters=channel,is_trigger,typeof_trigger,is_wakeup,wakeup_level  SFunctionDeploymentMode=off  EnableBusSupport=off  mask(MUXlink I/O Digital Input){channel=9, is_trigger=off, typeof_trigger=Either, is_wakeup=off, wakeup_level=Low level}
      mask prompts: channel "Channel ?"; is_trigger "Trigger ?"; typeof_trigger "Type of Trigger ?"; is_wakeup "Wake-up ?"; wakeup_level "Wake-up level ?"
      mask help: Read digital input from I/O channel.
      mask init:
      | NsiIo_DigitalInput_InitializationFcn();
      settings: OpenFcn=NsiIo_DigitalInput_OpenFcn();
      mask Help:
      | eval('block=get_param(gcb, ''RTWdata'');')
      | web([docroot '\toolbox\MUXlink\html\blocks/' block.MUXlink_BlockType '.html'])
      mask Callback channel: NsiIo_DigitalInput_ApplyFcn(1);
      mask Callback is_trigger: NsiIo_DigitalInput_ApplyFcn(2);
      mask TypeOptions typeof_trigger: Rising | Falling | Either
      mask Callback typeof_trigger: NsiIo_DigitalInput_ApplyFcn(3);
      mask Callback is_wakeup: NsiIo_DigitalInput_ApplyFcn(4);
      mask TypeOptions wakeup_level: Low level | High level
      mask Callback wakeup_level: NsiIo_DigitalInput_ApplyFcn(5);
      mask Display: image(imread('nsi.bmp'));text(0.5, 0.2, 'DigitalInput_9', 'horizontalAlignment', 'center', 'verticalAlignment', 'base');plot([0.05 0.05 0.05 0.05 0.05 0.05 0.05 0.05 0.05 0.05]);port_label('output', 1, 'Battery : C1');
  DigitalInput6 : S-Function  FunctionName=NsiIo_DigitalInput  Parameters=channel,is_trigger,typeof_trigger,is_wakeup,wakeup_level  SFunctionDeploymentMode=off  EnableBusSupport=off  mask(MUXlink I/O Digital Input){channel=10, is_trigger=off, typeof_trigger=Either, is_wakeup=off, wakeup_level=Low level}
      mask prompts: channel "Channel ?"; is_trigger "Trigger ?"; typeof_trigger "Type of Trigger ?"; is_wakeup "Wake-up ?"; wakeup_level "Wake-up level ?"
      mask help: Read digital input from I/O channel.
      mask init:
      | NsiIo_DigitalInput_InitializationFcn();
      settings: OpenFcn=NsiIo_DigitalInput_OpenFcn();
      mask Help:
      | eval('block=get_param(gcb, ''RTWdata'');')
      | web([docroot '\toolbox\MUXlink\html\blocks/' block.MUXlink_BlockType '.html'])
      mask Callback channel: NsiIo_DigitalInput_ApplyFcn(1);
      mask Callback is_trigger: NsiIo_DigitalInput_ApplyFcn(2);
      mask TypeOptions typeof_trigger: Rising | Falling | Either
      mask Callback typeof_trigger: NsiIo_DigitalInput_ApplyFcn(3);
      mask Callback is_wakeup: NsiIo_DigitalInput_ApplyFcn(4);
      mask TypeOptions wakeup_level: Low level | High level
      mask Callback wakeup_level: NsiIo_DigitalInput_ApplyFcn(5);
      mask Display: image(imread('nsi.bmp'));text(0.5, 0.2, 'DigitalInput_10', 'horizontalAlignment', 'center', 'verticalAlignment', 'base');plot([0.05 0.05 0.05 0.05 0.05 0.05 0.05 0.05 0.05 0.05]);port_label('output', 1, 'Battery : C2');
  btnRTD_Input : Outport
  btnX_Input : Outport  Port=2
  btnY_Input : Outport  Port=3
  btnZ_Input : Outport  Port=4
  btnPumpFan_Input : Outport  Port=5
  btnAccyFan_Input : Outport  Port=6
  wires:
  DigitalInput1/1 -> btnRTD_Input/1  "btnRTD_Input"
  DigitalInput4/1 -> btnY_Input/1  "btnY_Input"
  DigitalInput3/1 -> btnX_Input/1  "btnX_Input"
  DigitalInput2/1 -> btnZ_Input/1  "btnZ_Input"
  DigitalInput5/1 -> btnPumpFan_Input/1  "btnPumpFan_Input"
  DigitalInput6/1 -> btnAccyFan_Input/1  "btnAccyFan_Input"

== system TBRe19_ECU_SequentialTests/DriveFunction/Comms_And_Data_Acquisition_Layer/Hardwired_Inputs_2019/Pedal_Box ==
  AnalogInput1 : S-Function  FunctionName=NsiIo_AnalogInput  Parameters=channel  SFunctionDeploymentMode=off  EnableBusSupport=off  mask(MUXlink I/O Analog Input){channel=1, RANGE=0 / 20 Volts}
      mask prompts: channel "Channel ?"; RANGE "Plage de mesure"
      mask help: This block interface one of the 8 Analog Inputs. The analog inputs must be in the 0/20V range. Voltage output port provide a value in mV
      mask init:
      | NsiIo_AnalogInput_InitializationFcn();
      settings: OpenFcn=NsiIo_AnalogInput_OpenFcn();
      mask Help:
      | eval('block=get_param(gcb, ''RTWdata'');')
      | web([docroot '\toolbox\MUXlink\html\blocks/' block.MUXlink_BlockType '.html'])
      mask Callback channel: NsiIo_AnalogInput_ApplyFcn();
      mask Callback RANGE: NsiIo_AnalogInput_ApplyFcn();
      mask Display: image(imread('nsi.bmp'));text(0.5, 0.2, 'AnalogInput_1\n\n0 / 20 Volts', 'horizontalAlignment', 'center', 'verticalAlignment', 'base');plot([0.05 0.05 0.05 0.05 0.05 0.05 0.05 0.05 0.05 0.05]);port_label('output', 1, 'B1');
  AnalogInput2 : S-Function  FunctionName=NsiIo_AnalogInput  Parameters=channel  SFunctionDeploymentMode=off  EnableBusSupport=off  mask(MUXlink I/O Analog Input){channel=3, RANGE=0 / 20 Volts}
      mask prompts: channel "Channel ?"; RANGE "Plage de mesure"
      mask help: This block interface one of the 8 Analog Inputs. The analog inputs must be in the 0/20V range. Voltage output port provide a value in mV
      mask init:
      | NsiIo_AnalogInput_InitializationFcn();
      settings: OpenFcn=NsiIo_AnalogInput_OpenFcn();
      mask Help:
      | eval('block=get_param(gcb, ''RTWdata'');')
      | web([docroot '\toolbox\MUXlink\html\blocks/' block.MUXlink_BlockType '.html'])
      mask Callback channel: NsiIo_AnalogInput_ApplyFcn();
      mask Callback RANGE: NsiIo_AnalogInput_ApplyFcn();
      mask Display: image(imread('nsi.bmp'));text(0.5, 0.2, 'AnalogInput_3\n\n0 / 20 Volts', 'horizontalAlignment', 'center', 'verticalAlignment', 'base');plot([0.05 0.05 0.05 0.05 0.05 0.05 0.05 0.05 0.05 0.05]);port_label('output', 1, 'B3');
  AnalogInput3 : S-Function  FunctionName=NsiIo_AnalogInput  Parameters=channel  SFunctionDeploymentMode=off  EnableBusSupport=off  mask(MUXlink I/O Analog Input){channel=4, RANGE=0 / 20 Volts}
      mask prompts: channel "Channel ?"; RANGE "Plage de mesure"
      mask help: This block interface one of the 8 Analog Inputs. The analog inputs must be in the 0/20V range. Voltage output port provide a value in mV
      mask init:
      | NsiIo_AnalogInput_InitializationFcn();
      settings: OpenFcn=NsiIo_AnalogInput_OpenFcn();
      mask Help:
      | eval('block=get_param(gcb, ''RTWdata'');')
      | web([docroot '\toolbox\MUXlink\html\blocks/' block.MUXlink_BlockType '.html'])
      mask Callback channel: NsiIo_AnalogInput_ApplyFcn();
      mask Callback RANGE: NsiIo_AnalogInput_ApplyFcn();
      mask Display: image(imread('nsi.bmp'));text(0.5, 0.2, 'AnalogInput_4\n\n0 / 20 Volts', 'horizontalAlignment', 'center', 'verticalAlignment', 'base');plot([0.05 0.05 0.05 0.05 0.05 0.05 0.05 0.05 0.05 0.05]);port_label('output', 1, 'B4');
  AnalogInput6 : S-Function  FunctionName=NsiIo_AnalogInput  Parameters=channel  SFunctionDeploymentMode=off  EnableBusSupport=off  mask(MUXlink I/O Analog Input){channel=2, RANGE=0 / 20 Volts}
      mask prompts: channel "Channel ?"; RANGE "Plage de mesure"
      mask help: This block interface one of the 8 Analog Inputs. The analog inputs must be in the 0/20V range. Voltage output port provide a value in mV
      mask init:
      | NsiIo_AnalogInput_InitializationFcn();
      settings: OpenFcn=NsiIo_AnalogInput_OpenFcn();
      mask Help:
      | eval('block=get_param(gcb, ''RTWdata'');')
      | web([docroot '\toolbox\MUXlink\html\blocks/' block.MUXlink_BlockType '.html'])
      mask Callback channel: NsiIo_AnalogInput_ApplyFcn();
      mask Callback RANGE: NsiIo_AnalogInput_ApplyFcn();
      mask Display: image(imread('nsi.bmp'));text(0.5, 0.2, 'AnalogInput_2\n\n0 / 20 Volts', 'horizontalAlignment', 'center', 'verticalAlignment', 'base');plot([0.05 0.05 0.05 0.05 0.05 0.05 0.05 0.05 0.05 0.05]);port_label('output', 1, 'B2');
  AnalogInput7 : S-Function  FunctionName=NsiIo_AnalogInput  Parameters=channel  SFunctionDeploymentMode=off  EnableBusSupport=off  mask(MUXlink I/O Analog Input){channel=6, RANGE=0 / 20 Volts}
      mask prompts: channel "Channel ?"; RANGE "Plage de mesure"
      mask help: This block interface one of the 8 Analog Inputs. The analog inputs must be in the 0/20V range. Voltage output port provide a value in mV
      mask init:
      | NsiIo_AnalogInput_InitializationFcn();
      settings: OpenFcn=NsiIo_AnalogInput_OpenFcn();
      mask Help:
      | eval('block=get_param(gcb, ''RTWdata'');')
      | web([docroot '\toolbox\MUXlink\html\blocks/' block.MUXlink_BlockType '.html'])
      mask Callback channel: NsiIo_AnalogInput_ApplyFcn();
      mask Callback RANGE: NsiIo_AnalogInput_ApplyFcn();
      mask Display: image(imread('nsi.bmp'));text(0.5, 0.2, 'AnalogInput_6\n\n0 / 20 Volts', 'horizontalAlignment', 'center', 'verticalAlignment', 'base');plot([0.05 0.05 0.05 0.05 0.05 0.05 0.05 0.05 0.05 0.05]);port_label('output', 1, 'C4');
  Throttle1_Voltage : Outport
  Throttle2_Voltage : Outport  Port=2
  Brake_Voltage : Outport  Port=3
  Brake1_Pressure : Outport  Port=4
  Brake2_Pressure : Outport  Port=5
  wires:
  AnalogInput6/1 -> Throttle2_Voltage/1  "Throttle2_Voltage"
  AnalogInput1/1 -> Throttle1_Voltage/1  "Throttle1_Voltage"
  AnalogInput7/1 -> Brake_Voltage/1  "Brake_POT"
  AnalogInput2/1 -> Brake1_Pressure/1  "Brake1_Pressure"
  AnalogInput3/1 -> Brake2_Pressure/1  "Brake2_Pressure"
